simulink model "MBNLC_cascade_rov"  (Simulink 6.0)
settings: Solver=ode45  StartTime=0.0  StopTime=650  RelTol=1e-3
undefined symbols (not defined in the file): B, DQ, DQL, I, m, M, Ma, MaL, MaU, rg, sigbuilder_block, T, W, xb, xg, Xudot, yb, yg, Yvdot, zb, zg, Zwdot
libraries: simulink_extras x12, simulink x8
(part 1 of 3)
settings Model: LastModifiedBy=c chin

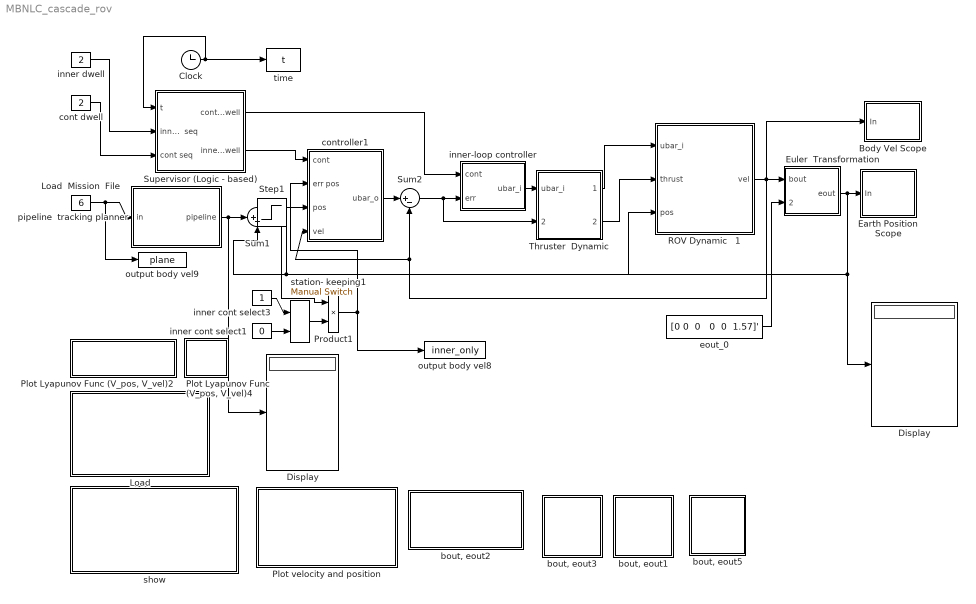
== system MBNLC_cascade_rov ==
  " Load  " : Subsystem  AncestorBlock=|
      | rov_design_analysis/ROV Controller
      | Design
      | Applications/ Load RRCROV2 parameters
      settings: OpenFcn=|
      | clc
      | cd c:\Matlab7\toolbox\rov_design_analysis\\mat_file ;
      | load rrcrovf;
      mask Display: disp('Double-click \n to \n Load the\n RRCROV\n parameters')
  " ROV Dynamic   1" : Subsystem
      mask Display:
      | disp('ROV')
      | image(imread('/rov_design_analysis/fig/ROVRRC2.jpg'));
      | color('white');port_label('input',1,'ubar_i')
      | color('white');port_label('input',2,'thrust')
      | color('white');port_label('input',3,'eout')
      | 
      | 
      | color('white');port_label('output',1,'vel')
  " inner dwell" : Constant  Value=2
  " station- keeping1" : simulink/Signal Routing/Manual Switch  sw=1  action=0
  Body Vel Scope : Subsystem  AncestorBlock=|
      | rov_design_analysis/ROV Controller
      | Design
      | Applications/1. Heading autopilot/Earth Position
      | Scope
      mask Display: disp('Body\nVelocity\nScope')
  Clock : Clock
      settings: Decimation=10
  Display : Display
  "Display  " : Display
  "Earth Position Scope " : Subsystem  AncestorBlock=|
      | rov_design_analysis/ROV Controller
      | Design
      | Applications/1. Heading autopilot/Earth Position
      | Scope
      mask Display: disp('Earth\nPosition\nScope')
  Euler  Transformation : Subsystem  AncestorBlock=rov_design_analysis/Scope Utilities/Euler Transformation
      mask Display: disp('Navigation \n Sensor')
  Load  Mission  File : Constant  Value=6
  "Plot Lyapunov Func (V_pos, V_vel)2" : Subsystem  AncestorBlock=|
      | rov_design_analysis/ROV Controller
      | Design
      | Applications/Plot velocity and position
      settings: OpenFcn=|
      | clc
      | close all
      mask Display: disp('Close All Figure')
  "Plot Lyapunov Func (V_pos, V_vel)4" : Subsystem  AncestorBlock=|
      | rov_design_analysis/ROV Controller
      | Design
      | Applications/Plot velocity and position
      settings: OpenFcn=|
      | clc
      | clear
      mask Display: disp('Clear')
  Plot velocity and position : Subsystem  AncestorBlock=|
      | rov_design_analysis/ROV Controller
      | Design
      | Applications/Plot velocity and position
      settings: OpenFcn=|
      | clc
      | cd c:\Matlab7\toolbox\rov_design_analysis\\m_file ;
      | run nonlin_resp6
      mask Display: disp('Double-click \n to \n Plot Velocity \n and \n Position')
  Product1 : Product  RndMeth=Zero
  Sum1 : Sum  Inputs=|+-  OutDataTypeMode=double  SaturateOnIntegerOverflow=on
  Sum2 : Sum  Inputs=|+-  OutDataTypeMode=double  SaturateOnIntegerOverflow=on
  Supervisor (Logic - based) : Subsystem
      mask Display: disp('Supervisor \n (Logic-based)')
  Thruster  Dynamic : Subsystem
      mask Display: disp('Thruster \n Dynamic')
  "bout, eout1" : Subsystem  AncestorBlock=|
      | rov_design_analysis/ROV Controller
      | Design
      | Applications/Plot velocity and position
      settings: OpenFcn=|
      | clc
      | cd c:\Matlab7\toolbox\rov_design_analysis\\m_file ;
      | figure
      | plot(eout(:,1),-eout(:,3))
      | xlabel('x')
      | ylabel('z')
      mask Display: disp('Plot \n XZ ')
  "bout, eout2" : Subsystem  AncestorBlock=|
      | rov_design_analysis/ROV Controller
      | Design
      | Applications/Plot velocity and position
      settings: OpenFcn=|
      | clc
      | cd c:\Matlab7\toolbox\rov_design_analysis\\m_file ;
      | figure
      | plot3(eout(:,1), eout(:,2),-eout(:,3))
      | xlabel('x')
      | ylabel('y')
      | zlabel('z')
      | grid on
      mask Display: disp('Plot \n 3D Response')
  "bout, eout3" : Subsystem  AncestorBlock=|
      | rov_design_analysis/ROV Controller
      | Design
      | Applications/Plot velocity and position
      settings: OpenFcn=|
      | clc
      | cd c:\Matlab7\toolbox\rov_design_analysis\\m_file ;
      | figure
      | plot(eout(:,1), eout(:,2))
      | xlabel('x')
      | ylabel('y')
      mask Display: disp('Plot \n XY ')
  "bout, eout5" : Subsystem  AncestorBlock=|
      | rov_design_analysis/ROV Controller
      | Design
      | Applications/Plot velocity and position
      settings: OpenFcn=|
      | clc
      | cd c:\Matlab7\toolbox\rov_design_analysis\\m_file ;
      | figure
      | box off
      | subplot(4,1,1)
      | plot(inner.time,inner.signals.values)
      | xlabel('time (sec)')
      | ylabel('Inner controller type')
      | subplot(4,1,2)
      | plot(outer.time,outer.signals.values)
      | xlabel('time (sec)')
      | ylabel('Outer controller type')
      | subplot(4,1,3)
      | plot(plane.time,plane.signals.values)
      | xlabel('time (sec)')
      | ylabel('Input sequence')
      | 
      | subplot(4,1,4)
      | plot(inner_only.time,inner_only.signals.values)
      | xlabel('time (sec)')
      | ylabel('Inner/Outer loop')
      mask Display: disp('Plot \n switching \n signal ')
  cont dwell : Constant  Value=2
  controller1 : Subsystem  Description=f(x)  AncestorBlock=|
      | rov_design_analysis/ROV Controller
      | Design
      | Applications/1. Heading autopilot/controller
      mask Display: disp('Nonlinear \n Model-Based \n Outer \n Controller')
  eout_0 : Constant  Value="[0 0  0   0  0  1.57]'"  OutDataTypeMode=double
  inner cont select1 : Constant  Value=0
  inner cont select3 : Constant
  inner-loop controller : Subsystem  Description=f(x)  AncestorBlock=|
      | rov_design_analysis/ROV Controller
      | Design
      | Applications/1. Heading autopilot/controller
      mask Display: disp('Inner Loop \n Controller')
  output body vel8 : ToWorkspace  VariableName=inner_only  SampleTime=1  SaveFormat=Structure With Time
  output body vel9 : ToWorkspace  VariableName=plane  SampleTime=1  SaveFormat=Structure With Time
  "pipeline  tracking planner  " : Subsystem  AncestorBlock=|
      | rov_design_analysis/ROV Controller
      | Design
      | Applications/1. Heading autopilot/pipe tracking
      | profile
      | (Auto)
      mask Display: disp('Pipeline Tracking \n Planner')
  show : Subsystem  AncestorBlock=|
      | rov_design_analysis/ROV Controller
      | Design
      | Applications/ Load RRCROV2 parameters
      settings: OpenFcn=|
      | clc
      | cd  c:\Matlab7\toolbox\rov_design_analysis\hybrid ;
      | open rrcrov2_para
      mask Display: disp('Double-click \n to \n SHOW\n RRCROV\n parameters')
  time : ToWorkspace  VariableName=t  SampleTime=1  SaveFormat=Array
  Step1 : Step  IOType=siggen  SampleTime=0
  wires:
  " ROV Dynamic   1"/1(vel) -> Body Vel Scope/1(In), Sum2/2, controller1/4(vel), Euler  Transformation/1(bout)
  Euler  Transformation/1(eout) -> "Earth Position Scope "/1(In), controller1/3(pos), Sum1/2, " ROV Dynamic   1"/3("pos "), "Display  "/1
  Clock/1 -> time/1, Supervisor (Logic - based)/1(t)
  Thruster  Dynamic/2(thruster_out) -> " ROV Dynamic   1"/2("thrust ")
  Sum2/1 -> Thruster  Dynamic/2(bout_err), inner-loop controller/2(err)
  Thruster  Dynamic/1(cont_out) -> " ROV Dynamic   1"/1(ubar_i)
  inner-loop controller/1(ubar_i) -> Thruster  Dynamic/1(ubar_i)
  "pipeline  tracking planner  "/1(pipeline) -> Sum1/1, Display/1
  Supervisor (Logic - based)/1(cont dwell) -> inner-loop controller/1(cont)
  controller1/1(ubar_o) -> Sum2/1
  " inner dwell"/1 -> Supervisor (Logic - based)/2(inner  seq)
  cont dwell/1 -> Supervisor (Logic - based)/3(cont seq)
  eout_0/1 -> Euler  Transformation/2(eout_0)
  Load  Mission  File/1 -> output body vel9/1, "pipeline  tracking planner  "/1(in)
  inner cont select3/1 -> " station- keeping1"/1
  inner cont select1/1 -> " station- keeping1"/2
  " station- keeping1"/1 -> Product1/2
  Sum1/1 -> Product1/1
  Supervisor (Logic - based)/2(inner  dwell) -> controller1/1(cont)
  Product1/1 -> controller1/2(err pos), output body vel8/1

== system MBNLC_cascade_rov/ Load   ==

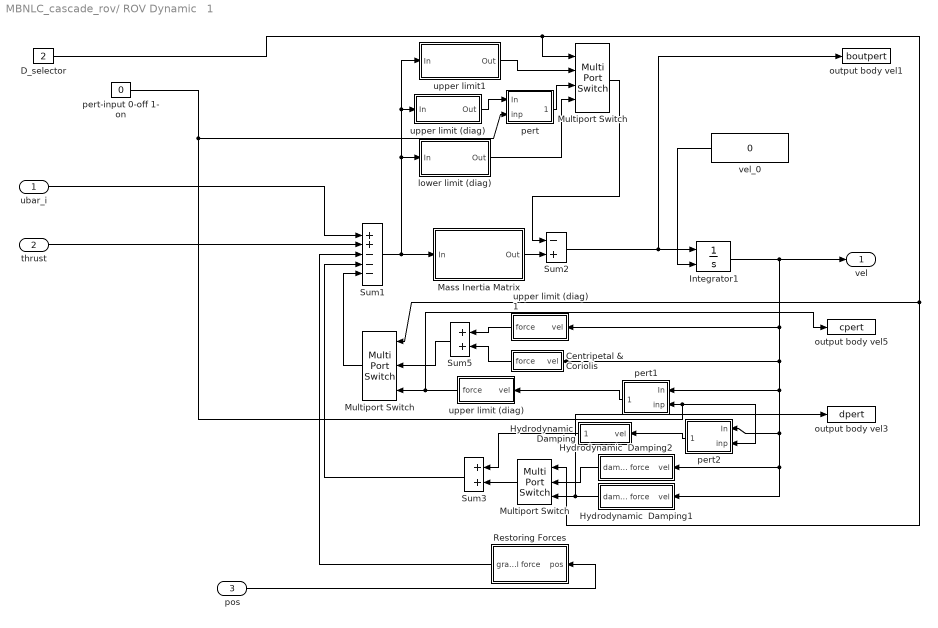
== system MBNLC_cascade_rov/ ROV Dynamic   1 ==
  ubar_i : Inport  Port=1  LatchInput=off
  "thrust " : Inport  Port=2  LatchInput=off
  "pos " : Inport  Port=3  LatchInput=off
  Centripetal & Coriolis : Subsystem  Orientation=left  AncestorBlock=rov_design_analysis/ROV Models/1. Six DOF RRC ROV II/Centripetal & Coriolis
      mask Display: disp('C')
  D_selector : Constant  Value=2
  Hydrodynamic  Damping : Subsystem  Orientation=left
      mask Display: disp('D')
  Hydrodynamic  Damping1 : Subsystem  Orientation=left
      mask Display: disp('perturb \nDamping')
  Hydrodynamic  Damping2 : Subsystem  Orientation=left
      mask Display: disp('Zero Perturb')
  Integrator1 : Integrator  InitialConditionSource=external
  Mass Inertia Matrix : Subsystem
      mask Display: disp('inv(MRB+MA)')
  Multiport Switch : MultiPortSwitch  Inputs=3
  "Multiport Switch  " : MultiPortSwitch  Orientation=left  Inputs=2
  "Multiport Switch    " : MultiPortSwitch  Orientation=left  Inputs=2
  Restoring Forces : Subsystem  Orientation=left
      mask Display: disp('Restoring\nForce')
  Sum1 : Sum  Inputs=++---  SaturateOnIntegerOverflow=on  InputSameDT=on
  Sum2 : Sum  Inputs=-+  SaturateOnIntegerOverflow=on  InputSameDT=on
  Sum3 : Sum  Orientation=left  SaturateOnIntegerOverflow=on  InputSameDT=on
  Sum5 : Sum  Orientation=left  SaturateOnIntegerOverflow=on  InputSameDT=on
  lower limit (diag) : Subsystem
      mask Display: disp('Perturb MA')
  output body vel1 : ToWorkspace  VariableName=boutpert  SampleTime=1  SaveFormat=Array
  output body vel3 : ToWorkspace  VariableName=dpert  SampleTime=1  SaveFormat=Array
  output body vel5 : ToWorkspace  VariableName=cpert  SampleTime=1  SaveFormat=Array
  pert : Subsystem
  pert-input 0-off 1- on : Constant  Value=0
  pert1 : Subsystem  Orientation=left
  pert2 : Subsystem  Orientation=left
  upper limit (diag) : Subsystem
      mask Display: disp('Perturb MA')
  "upper limit (diag)   " : Subsystem  Orientation=left
      mask Display: disp('Perturb CA')
  upper limit (diag)   1 : Subsystem  Orientation=left
      mask Display: disp('CA')
  upper limit1 : Subsystem
      mask Display: disp('Zero Perturb')
  vel_0 : Constant  Orientation=left  Value=0  OutDataTypeMode=double
  vel : Outport
  wires:
  Restoring Forces/1(gravitational force) -> Sum1/3
  "thrust "/1 -> Sum1/2
  Sum1/1 -> Mass Inertia Matrix/1(In), upper limit1/1(In), upper limit (diag)/1(In), lower limit (diag)/1(In)
  "Multiport Switch  "/1 -> Sum1/5
  "pos "/1 -> Restoring Forces/1(pos)
  Mass Inertia Matrix/1(Out) -> Sum2/2
  upper limit1/1(Out) -> Multiport Switch/2
  lower limit (diag)/1(Out) -> Multiport Switch/4
  Multiport Switch/1 -> Sum2/1
  "upper limit (diag)   "/1(force) -> "Multiport Switch  "/3, output body vel5/1
  Sum5/1 -> "Multiport Switch  "/2
  Hydrodynamic  Damping1/1(damping force) -> "Multiport Switch    "/3, output body vel3/1
  Hydrodynamic  Damping2/1(damping force) -> "Multiport Switch    "/2
  Sum3/1 -> Sum1/4
  "Multiport Switch    "/1 -> Sum3/2
  Hydrodynamic  Damping/1(damping force) -> Sum3/1
  upper limit (diag)   1/1(force) -> Sum5/1
  Centripetal & Coriolis/1(force) -> Sum5/2
  Sum2/1 -> output body vel1/1, Integrator1/1
  Integrator1/1 -> vel/1, upper limit (diag)   1/1(vel), Centripetal & Coriolis/1(vel), Hydrodynamic  Damping1/1(vel), Hydrodynamic  Damping2/1(vel), pert2/1(In), pert1/1(In)
  vel_0/1 -> Integrator1/2
  ubar_i/1 -> Sum1/1
  pert2/1(on/off) -> Hydrodynamic  Damping/1(vel)
  pert1/1(on/off) -> "upper limit (diag)   "/1(vel)
  upper limit (diag)/1(Out) -> pert/1(In)
  pert/1(on/off) -> Multiport Switch/3
  pert-input 0-off 1- on/1 -> pert/2(inp), pert1/2(inp), pert2/2(inp)
  D_selector/1 -> Multiport Switch/1, "Multiport Switch  "/1, "Multiport Switch    "/1

== system MBNLC_cascade_rov/Body Vel Scope ==
  In : Inport  Port=1  LatchInput=off
  Demux : Demux  Outputs=6
  output body vel4 : ToWorkspace  VariableName=bout  SampleTime=1  SaveFormat=Array
  phi : Scope
      settings: TickLabels=on  YMin=-0.125  YMax=0.2  DataFormat=Array
  theta : Scope
      settings: TickLabels=on  TimeRange=200  YMin=-0.05  YMax=0.15  DataFormat=Array
  x : Scope
      settings: TickLabels=on  TimeRange=50  YMin=-0.025  YMax=0.375  DataFormat=Array
  y : Scope
      settings: TickLabels=on  YMin=-0.02  YMax=0.1  DataFormat=Array
  yaw : Scope
      settings: TickLabels=on  TimeRange=200  YMin=-0.05  YMax=0.15  SaveName=ScopeData2  DataFormat=Array
  z : Scope
      settings: TickLabels=on  TimeRange=50  YMin=-0.0025  YMax=0.0375  DataFormat=Array
  wires:
  Demux/5 -> theta/1
  In/1 -> Demux/1, output body vel4/1
  Demux/3 -> z/1
  Demux/4 -> phi/1
  Demux/2 -> y/1
  Demux/1 -> x/1
  Demux/6 -> yaw/1

== system MBNLC_cascade_rov/Earth Position Scope  ==
  In : Inport  Port=1  LatchInput=off
  Demux : Demux  Outputs=6
  XY Graph : simulink/Sinks/XY Graph  xmin=-50  xmax=50  ymin=-50  ymax=50  st=-1
  output body vel5 : ToWorkspace  VariableName=eout  SampleTime=1  SaveFormat=Array
  phi : Scope
      settings: TickLabels=on  YMin=-0.125  YMax=0.2  DataFormat=Array
  theta : Scope
      settings: TickLabels=on  TimeRange=200  YMin=-0.05  YMax=0.15  DataFormat=Array
  x : Scope
      settings: TickLabels=on  TimeRange=50  YMin=-0.025  YMax=0.375  DataFormat=Array
  y : Scope
      settings: TickLabels=on  YMin=-0.02  YMax=0.1  DataFormat=Array
  yaw : Scope
      settings: TickLabels=on  TimeRange=200  YMin=-0.05  YMax=0.15  SaveName=ScopeData2  DataFormat=Array
  z : Scope
      settings: TickLabels=on  TimeRange=50  YMin=-0.0025  YMax=0.0375  DataFormat=Array
  wires:
  Demux/5 -> theta/1
  In/1 -> Demux/1, output body vel5/1
  Demux/3 -> z/1
  Demux/4 -> phi/1
  Demux/2 -> y/1, XY Graph/2
  Demux/1 -> x/1, XY Graph/1
  Demux/6 -> yaw/1

== system MBNLC_cascade_rov/Euler  Transformation ==
  bout : Inport  Port=1  LatchInput=off
  eout_0 : Inport  Port=2  LatchInput=off
  Demux : Demux  Outputs=2
  Demux1 : Demux  Outputs=2
  Intregrator2 : Integrator  InitialConditionSource=external
  Mux1 : Mux  Inputs=2
  Terminator : Terminator
  Transformation matrix R : Subsystem
      mask Display: disp('Transformation R')
  Transformation matrix T : Subsystem
      mask Display: disp('Transformation T')
  output body vel1 : ToWorkspace  VariableName=eoutpert  SampleTime=1  SaveFormat=Array
  eout : Outport  InitialOutput=0
  wires:
  Mux1/1 -> Intregrator2/1
  Intregrator2/1 -> Demux1/1, eout/1, output body vel1/1
  Demux/2 -> Transformation matrix R/1(angular body  velocity)
  Demux/1 -> Transformation matrix T/1(translational body velocity)
  bout/1 -> Demux/1
  Demux1/2 -> Transformation matrix T/2(angular position), Transformation matrix R/2(angular position)
  Transformation matrix R/1(angular earth velocity) -> Mux1/2
  Transformation matrix T/1(translational earth velocity) -> Mux1/1
  Demux1/1 -> Terminator/1
  eout_0/1 -> Intregrator2/2

== system MBNLC_cascade_rov/Plot Lyapunov Func (V_pos, V_vel)2 ==

== system MBNLC_cascade_rov/Plot Lyapunov Func (V_pos, V_vel)4 ==

== system MBNLC_cascade_rov/Plot velocity and position ==

== system MBNLC_cascade_rov/Supervisor (Logic - based) ==
  t : Inport  Port=1  LatchInput=off
  inner  seq : Inport  Port=2  LatchInput=off
  cont seq : Inport  Port=3  LatchInput=off
  150-300 : Relay  OnSwitchValue=150  OffSwitchValue=0  OnOutputValue=0  OffOutputValue=1
  Constant1 : Constant
  Constant8 : Constant
  Switching sequence : Subsystem  AncestorBlock=rov_design_analysis/Scope Utilities/Switching sequence
      mask Display: disp('Dwell \n Sequence')
  Switching sequence1 : Subsystem  AncestorBlock=rov_design_analysis/Scope Utilities/Switching sequence
      mask Display: disp('Dwell \n Sequence')
  "cont dwell switch  " : MultiPortSwitch  Inputs=2
  inner dwell Switch : MultiPortSwitch  Inputs=3
  output body vel6 : ToWorkspace  VariableName=outer  SampleTime=1  SaveFormat=Structure With Time
  cont dwell : Outport
  inner  dwell : Outport  Port=2
  wires:
  inner  seq/1 -> inner dwell Switch/1
  150-300/1 -> inner dwell Switch/2  "1"
  Constant8/1 -> inner dwell Switch/3  "2"
  inner dwell Switch/1 -> inner  dwell/1
  cont seq/1 -> "cont dwell switch  "/1
  "cont dwell switch  "/1 -> cont dwell/1, output body vel6/1
  t/1 -> 150-300/1
  Switching sequence1/1(" ") -> "cont dwell switch  "/2
  Constant1/1 -> "cont dwell switch  "/3
  Switching sequence/1(" ") -> inner dwell Switch/4  "3"

== system MBNLC_cascade_rov/Thruster  Dynamic ==
  ubar_i : Inport  Port=1  LatchInput=off
  bout_err : Inport  Port=2  LatchInput=off
  Sum2 : Sum  Inputs=|++  OutDataTypeMode=double  SaturateOnIntegerOverflow=on
  Thruster configuration1 : Subsystem  AncestorBlock=|
      | rov_design_analysis/ROV Controller
      | Design
      | Applications/1. Heading autopilot/Thruster
      | configuration
      mask Display: disp('T')
  Thruster configuration2 : Subsystem  AncestorBlock=|
      | rov_design_analysis/ROV Controller
      | Design
      | Applications/1. Heading autopilot/Thruster
      | configuration
      mask Display: disp('Kc')
  Thruster configuration3 : Subsystem  AncestorBlock=|
      | rov_design_analysis/ROV Controller
      | Design
      | Applications/1. Heading autopilot/Thruster
      | configuration
      mask Display: disp('Kc')
  Thruster configuration4 : Subsystem  AncestorBlock=|
      | rov_design_analysis/ROV Controller
      | Design
      | Applications/1. Heading autopilot/Thruster
      | configuration
      mask Display: disp('T')
  output earth pos1 : ToWorkspace  VariableName=thrustdc  SampleTime=1  SaveFormat=Array
  output earth pos2 : ToWorkspace  VariableName=thrustd  SampleTime=1  SaveFormat=Array
  output earth pos3 : ToWorkspace  VariableName=thrust  SampleTime=1  SaveFormat=Array
  thruster  dynamic     1 : Subsystem
  cont_out : Outport
  thruster_out : Outport  Port=2
  wires:
  Thruster configuration1/1(output force) -> Thruster configuration2/1(input velocity)
  Thruster configuration4/1(output force) -> Thruster configuration3/1(input velocity)
  thruster  dynamic     1/1(T) -> Thruster configuration1/1(input velocity), Sum2/2, output earth pos3/1
  bout_err/1 -> thruster  dynamic     1/1(volt)
  Thruster configuration3/1(output force) -> cont_out/1
  ubar_i/1 -> Thruster configuration4/1(input velocity), Sum2/1, output earth pos1/1
  Thruster configuration2/1(output force) -> thruster_out/1
  Sum2/1 -> output earth pos2/1

== system MBNLC_cascade_rov/bout, eout1 ==

== system MBNLC_cascade_rov/bout, eout2 ==

== system MBNLC_cascade_rov/bout, eout3 ==

== system MBNLC_cascade_rov/bout, eout5 ==

== system MBNLC_cascade_rov/controller1 ==
  cont : Inport  Port=1  LatchInput=off
  err pos : Inport  Port=2  LatchInput=off
  pos : Inport  Port=3  LatchInput=off
  vel : Inport  Port=4  LatchInput=off
  Multiport Switch : MultiPortSwitch  Inputs=2
  Nonlinear model based  PD controller : Subsystem
  PD : Subsystem
  "boutd  " : Constant  Value="[0 0  0   0  0  0]'"  OutDataTypeMode=double
  ubar_o : Outport
  wires:
  Multiport Switch/1 -> ubar_o/1
  cont/1 -> Multiport Switch/1
  "boutd  "/1 -> Nonlinear model based  PD controller/2(vel_d)
  Nonlinear model based  PD controller/1(" ") -> Multiport Switch/2
  PD/1(" ") -> Multiport Switch/3
  err pos/1 -> PD/1(err), Nonlinear model based  PD controller/1(errpos)
  pos/1 -> Nonlinear model based  PD controller/3(pos)
  vel/1 -> Nonlinear model based  PD controller/4(vel)

== system MBNLC_cascade_rov/inner-loop controller ==
  cont : Inport  Port=1  LatchInput=off
  err : Inport  Port=2  LatchInput=off
  MCD_selector : Constant  Value=2
  Multiport Switch : MultiPortSwitch
  "inner -PI-decouple " : Subsystem
  inner -backstepping : Subsystem
  inner-P : Subsystem
  inner-sliding : Subsystem
  output body vel7 : ToWorkspace  VariableName=inner  SampleTime=1  SaveFormat=Structure With Time
  ubar_i : Outport
  wires:
  Multiport Switch/1 -> ubar_i/1
  cont/1 -> Multiport Switch/1, output body vel7/1
  "inner -PI-decouple "/1(" ") -> Multiport Switch/2
  inner-P/1(" ") -> Multiport Switch/3
  err/1 -> inner-P/1(P), inner-sliding/1(sliding), inner -backstepping/1(err), "inner -PI-decouple "/1(err)
  inner -backstepping/1(" ") -> Multiport Switch/4
  inner-sliding/1(" ") -> Multiport Switch/5
  MCD_selector/1 -> inner -backstepping/2(M_select)

== system MBNLC_cascade_rov/pipeline  tracking planner   ==
  in : Inport  Port=1  LatchInput=off
  decoupled input : Subsystem
  pipeline : Outport
  wires:
  in/1 -> decoupled input/1(In1)
  decoupled input/1(Out1) -> pipeline/1

== system MBNLC_cascade_rov/show ==

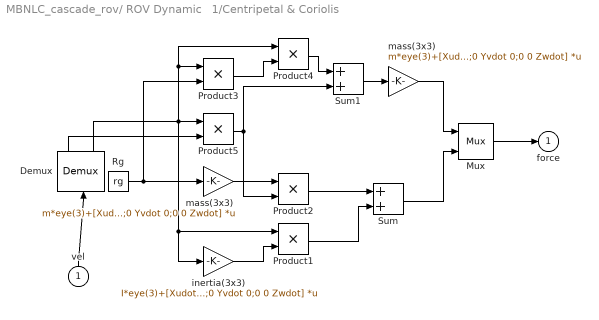
== system MBNLC_cascade_rov/ ROV Dynamic   1/Centripetal & Coriolis ==
  vel : Inport  Orientation=up  Port=1  LatchInput=off
  Demux : Demux  Orientation=up  Outputs=2
  Mux : Mux  Inputs=2
  Product{1..5} (5 alike) : Product  SaturateOnIntegerOverflow=on  RndMeth=Zero  InputSameDT=on
  Rg : Constant  Value=rg
  Sum : Sum  SaturateOnIntegerOverflow=on  InputSameDT=on
  Sum1 : Sum  SaturateOnIntegerOverflow=on  InputSameDT=on
  inertia(3x3) : Gain  Gain=I*eye(3)+[Xudot 0 0;0 Yvdot 0;0 0 Zwdot]  Multiplication=Matrix(K*u)  SaturateOnIntegerOverflow=on
  "mass(3x3) " : Gain  Gain=m*eye(3)+[Xudot 0 0;0 Yvdot 0;0 0 Zwdot]  Multiplication=Matrix(K*u)  SaturateOnIntegerOverflow=on
  "mass(3x3)   " : Gain  Gain=m*eye(3)+[Xudot 0 0;0 Yvdot 0;0 0 Zwdot]  Multiplication=Matrix(K*u)  SaturateOnIntegerOverflow=on
  force : Outport  InitialOutput=0
  wires:
  Product1/1 -> Sum/2
  "mass(3x3)   "/1 -> Product2/1
  Product2/1 -> Sum/1
  Rg/1 -> Product3/2, "mass(3x3)   "/1
  Product3/1 -> Product4/2
  Product4/1 -> Sum1/1
  Product5/1 -> Product2/2, Sum1/2
  Sum1/1 -> "mass(3x3) "/1
  Demux/2 -> Product5/1, Product3/1, Product4/1, Product1/1, inertia(3x3)/1
  Demux/1 -> Product5/2
  vel/1 -> Demux/1
  inertia(3x3)/1 -> Product1/2
  "mass(3x3) "/1 -> Mux/1
  Sum/1 -> Mux/2
  Mux/1 -> force/1

== system MBNLC_cascade_rov/ ROV Dynamic   1/Hydrodynamic  Damping ==
  vel : Inport  Port=1  LatchInput=off
  D linear : Gain  Gain=-diag(DQL)  SaturateOnIntegerOverflow=on
  damping force : Outport  InitialOutput=0
  wires:
  vel/1 -> D linear/1
  D linear/1 -> damping force/1

== system MBNLC_cascade_rov/ ROV Dynamic   1/Hydrodynamic  Damping1 ==
  vel : Inport  Port=1  LatchInput=off
  D quadratic : Gain  Gain=-diag(DQ)  SaturateOnIntegerOverflow=on
  Product : Product  SaturateOnIntegerOverflow=on  RndMeth=Zero  InputSameDT=on
  |u| : Abs  SaturateOnIntegerOverflow=on
  damping force : Outport  InitialOutput=0
  wires:
  Product/1 -> D quadratic/1
  vel/1 -> Product/1, |u|/1
  |u|/1 -> Product/2
  D quadratic/1 -> damping force/1

== system MBNLC_cascade_rov/ ROV Dynamic   1/Hydrodynamic  Damping2 ==
  vel : Inport  Port=1  LatchInput=off
  D quadratic : Gain  Gain=0  SaturateOnIntegerOverflow=on
  damping force : Outport  InitialOutput=0
  wires:
  D quadratic/1 -> damping force/1
  vel/1 -> D quadratic/1

== system MBNLC_cascade_rov/ ROV Dynamic   1/Mass Inertia Matrix ==
  In : Inport  Port=1  LatchInput=off
  inverse M : Gain  Gain=inv(M-Ma)  Multiplication=Matrix(K*u)  SaturateOnIntegerOverflow=on
  Out : Outport
  wires:
  inverse M/1 -> Out/1
  In/1 -> inverse M/1

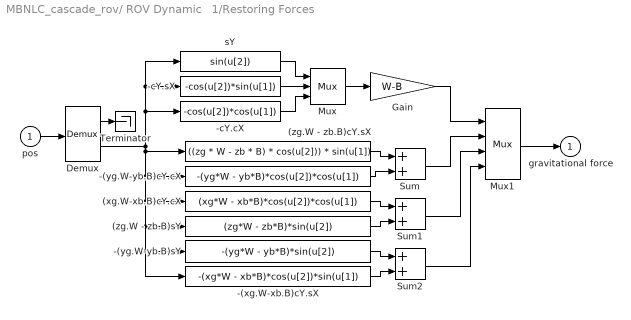
== system MBNLC_cascade_rov/ ROV Dynamic   1/Restoring Forces ==
  pos : Inport  Port=1  LatchInput=off
  (xg.W-xb.B)cY.cX : Fcn  Expr=(xg*W - xb*B)*cos(u[2])*cos(u[1])
  (zg.W - zb.B)cY.sX : Fcn  Expr=((zg * W - zb * B) * cos(u[2])) * sin(u[1])
  (zg.W - zb.B)sY : Fcn  Expr=(zg*W - zb*B)*sin(u[2])
  -(xg.W-xb.B)cY.sX : Fcn  Expr=-(xg*W - xb*B)*cos(u[2])*sin(u[1])
  -(yg.W-yb.B)cY.cX : Fcn  Expr=-(yg*W - yb*B)*cos(u[2])*cos(u[1])
  -(yg.W-yb.B)sY : Fcn  Expr=-(yg*W - yb*B)*sin(u[2])
  -cY.cX : Fcn  Expr=-cos(u[2])*cos(u[1])
  -cY.sX : Fcn  Expr=-cos(u[2])*sin(u[1])
  Demux : Demux  Outputs=2
  Gain : Gain  Gain=W-B  SaturateOnIntegerOverflow=on
  Mux : Mux  Inputs=3
  Mux1 : Mux
  Sum : Sum  SaturateOnIntegerOverflow=on  InputSameDT=on
  Sum1 : Sum  SaturateOnIntegerOverflow=on  InputSameDT=on
  Sum2 : Sum  SaturateOnIntegerOverflow=on  InputSameDT=on
  Terminator : Terminator
  sY : Fcn  Expr=sin(u[2])
  gravitational force : Outport  InitialOutput=0
  wires:
  Sum2/1 -> Mux1/4
  -(yg.W-yb.B)sY/1 -> Sum2/1
  -(xg.W-xb.B)cY.sX/1 -> Sum2/2
  Sum1/1 -> Mux1/3
  (xg.W-xb.B)cY.cX/1 -> Sum1/1
  (zg.W - zb.B)sY/1 -> Sum1/2
  Sum/1 -> Mux1/2
  (zg.W - zb.B)cY.sX/1 -> Sum/1
  -(yg.W-yb.B)cY.cX/1 -> Sum/2
  Gain/1 -> Mux1/1
  Mux/1 -> Gain/1
  -cY.cX/1 -> Mux/3
  -cY.sX/1 -> Mux/2
  sY/1 -> Mux/1
  Mux1/1 -> gravitational force/1
  Demux/2 -> -(xg.W-xb.B)cY.sX/1, -(yg.W-yb.B)sY/1, (zg.W - zb.B)sY/1, (xg.W-xb.B)cY.cX/1, -(yg.W-yb.B)cY.cX/1, (zg.W - zb.B)cY.sX/1, sY/1, -cY.sX/1, -cY.cX/1
  Demux/1 -> Terminator/1
  pos/1 -> Demux/1

== system MBNLC_cascade_rov/ ROV Dynamic   1/lower limit (diag) ==
  In : Inport  Port=1  LatchInput=off
  inverse M : Gain  Gain=-diag([21.1403-21.0981 51.7012-51.0026 92.451-91.837 3.6191-3.576 2.6427-2.7687 2.3033-2.3493])  Multiplication=Matrix(K*u)  SaturateOnIntegerOverflow=on
  Out : Outport
  wires:
  inverse M/1 -> Out/1
  In/1 -> inverse M/1

== system MBNLC_cascade_rov/ ROV Dynamic   1/pert ==
  In : Inport  Port=1  LatchInput=off
  inp : Inport  Port=2  LatchInput=off
  D linear3 : Gain  Gain=2  SaturateOnIntegerOverflow=on
  Product : Product  RndMeth=Zero
  Sine Wave-pert : Sin  Amplitude=0.1  SampleTime=0
  Sum6 : Sum  Inputs=|++  SaturateOnIntegerOverflow=on  InputSameDT=on
  on/off : Outport
  wires:
  D linear3/1 -> Sum6/1
  Sine Wave-pert/1 -> Product/1
  Product/1 -> Sum6/2
  inp/1 -> Product/2
  In/1 -> D linear3/1
  Sum6/1 -> on/off/1

== system MBNLC_cascade_rov/ ROV Dynamic   1/pert1 ==
  In : Inport  Port=1  LatchInput=off
  inp : Inport  Port=2  LatchInput=off
  D linear3 : Gain  Gain=2  SaturateOnIntegerOverflow=on
  Product : Product  RndMeth=Zero
  Sine Wave-pert : Sin  Amplitude=0.1  SampleTime=0
  Sum6 : Sum  Inputs=|++  SaturateOnIntegerOverflow=on  InputSameDT=on
  on/off : Outport
  wires:
  D linear3/1 -> Sum6/1
  Sine Wave-pert/1 -> Product/1
  Product/1 -> Sum6/2
  inp/1 -> Product/2
  In/1 -> D linear3/1
  Sum6/1 -> on/off/1

== system MBNLC_cascade_rov/ ROV Dynamic   1/pert2 ==
  In : Inport  Port=1  LatchInput=off
  inp : Inport  Port=2  LatchInput=off
  D linear3 : Gain  Gain=2  SaturateOnIntegerOverflow=on
  Product : Product  RndMeth=Zero
  Sine Wave-pert : Sin  Amplitude=0.1  SampleTime=0
  Sum6 : Sum  Inputs=|++  SaturateOnIntegerOverflow=on  InputSameDT=on
  on/off : Outport
  wires:
  D linear3/1 -> Sum6/1
  Sine Wave-pert/1 -> Product/1
  Product/1 -> Sum6/2
  inp/1 -> Product/2
  In/1 -> D linear3/1
  Sum6/1 -> on/off/1

== system MBNLC_cascade_rov/ ROV Dynamic   1/upper limit (diag) ==
  In : Inport  Port=1  LatchInput=off
  inverse M : Gain  Gain=-diag([21.724-21.1403 51.7013-51.7012 94.3-92.451 4.2176-3.6191 7.1148-2.6427 4.7673-2.3033])  Multiplication=Matrix(K*u)  SaturateOnIntegerOverflow=on
  Out : Outport
  wires:
  inverse M/1 -> Out/1
  In/1 -> inverse M/1

== system MBNLC_cascade_rov/ ROV Dynamic   1/upper limit (diag)    ==
  note: 7 8 9 10 11 12
  note: 1 2 3 4 5 6
  vel : Inport  Port=1  LatchInput=off
  (zg.W - zb.B)cY.sX : Fcn  Expr=-u[9]*u[3]*u[5]+u[8]*u[2]*u[6]
  (zg.W - zb.B)cY.sX1 : Fcn  Expr=u[9]*u[3]*u[4]-u[7]*u[1]*u[6]
  (zg.W - zb.B)cY.sX2 : Fcn  Expr=-u[8]*u[2]*u[4]+u[7]*u[1]*u[5]
  (zg.W - zb.B)cY.sX3 : Fcn  Expr=-u[9]*u[3]*u[2]+u[8]*u[2]*u[3]-u[12]*u[6]*u[5]+u[11]*u[5]*u[6]
  (zg.W - zb.B)cY.sX4 : Fcn  Expr=u[9]*u[3]*u[1]-u[7]*u[1]*u[3]+u[6]*u[12]*u[4]-u[4]*u[10]*u[6]
  (zg.W - zb.B)cY.sX5 : Fcn  Expr=-u[8]*u[2]*u[1]+u[7]*u[1]*u[2]-u[11]*u[5]*u[4]+u[10]*u[4]*u[5]
  Mux1 : Mux  Inputs=6
  Mux3 : Mux  Inputs=2
  Rg1 : Constant  Value="[MaU(1)  MaU(2)  MaU(3)  MaU(4)  MaU(5)  MaU(6) ]'"
  force : Outport
  wires:
  Mux1/1 -> force/1
  (zg.W - zb.B)cY.sX/1 -> Mux1/1
  (zg.W - zb.B)cY.sX1/1 -> Mux1/2
  (zg.W - zb.B)cY.sX2/1 -> Mux1/3
  (zg.W - zb.B)cY.sX3/1 -> Mux1/4
  (zg.W - zb.B)cY.sX4/1 -> Mux1/5
  (zg.W - zb.B)cY.sX5/1 -> Mux1/6
  vel/1 -> Mux3/1
  Rg1/1 -> Mux3/2
  Mux3/1 -> (zg.W - zb.B)cY.sX/1, (zg.W - zb.B)cY.sX1/1, (zg.W - zb.B)cY.sX4/1, (zg.W - zb.B)cY.sX5/1, (zg.W - zb.B)cY.sX3/1, (zg.W - zb.B)cY.sX2/1

== system MBNLC_cascade_rov/ ROV Dynamic   1/upper limit (diag)   1 ==
  note: 7 8 9 10 11 12
  note: 1 2 3 4 5 6
  vel : Inport  Port=1  LatchInput=off
  (zg.W - zb.B)cY.sX : Fcn  Expr=-u[9]*u[3]*u[5]+u[8]*u[2]*u[6]
  (zg.W - zb.B)cY.sX1 : Fcn  Expr=u[9]*u[3]*u[4]-u[7]*u[1]*u[6]
  (zg.W - zb.B)cY.sX2 : Fcn  Expr=-u[8]*u[2]*u[4]+u[7]*u[1]*u[5]
  (zg.W - zb.B)cY.sX3 : Fcn  Expr=-u[9]*u[3]*u[2]+u[8]*u[2]*u[3]-u[12]*u[6]*u[5]+u[11]*u[5]*u[6]
  (zg.W - zb.B)cY.sX4 : Fcn  Expr=u[9]*u[3]*u[1]-u[7]*u[1]*u[3]+u[6]*u[12]*u[4]-u[4]*u[10]*u[6]
  (zg.W - zb.B)cY.sX5 : Fcn  Expr=-u[8]*u[2]*u[1]+u[7]*u[1]*u[2]-u[11]*u[5]*u[4]+u[10]*u[4]*u[5]
  Mux1 : Mux  Inputs=6
  Mux3 : Mux  Inputs=2
  Rg1 : Constant  Value="[Ma(1)  Ma(2)  Ma(3)  Ma(4)  Ma(5)  Ma(6) ]'"
  force : Outport
  wires:
  Mux1/1 -> force/1
  (zg.W - zb.B)cY.sX/1 -> Mux1/1
  (zg.W - zb.B)cY.sX1/1 -> Mux1/2
  (zg.W - zb.B)cY.sX2/1 -> Mux1/3
  (zg.W - zb.B)cY.sX3/1 -> Mux1/4
  (zg.W - zb.B)cY.sX4/1 -> Mux1/5
  (zg.W - zb.B)cY.sX5/1 -> Mux1/6
  vel/1 -> Mux3/1
  Rg1/1 -> Mux3/2
  Mux3/1 -> (zg.W - zb.B)cY.sX/1, (zg.W - zb.B)cY.sX1/1, (zg.W - zb.B)cY.sX4/1, (zg.W - zb.B)cY.sX5/1, (zg.W - zb.B)cY.sX3/1, (zg.W - zb.B)cY.sX2/1

== system MBNLC_cascade_rov/ ROV Dynamic   1/upper limit1 ==
  In : Inport  Port=1  LatchInput=off
  inverse M : Gain  Gain=0  Multiplication=Matrix(K*u)  SaturateOnIntegerOverflow=on
  Out : Outport
  wires:
  inverse M/1 -> Out/1
  In/1 -> inverse M/1

== system MBNLC_cascade_rov/Euler  Transformation/Transformation matrix R ==
  angular body  velocity : Inport  Port=1  LatchInput=off
  angular position : Inport  Port=2  LatchInput=off
  Mux : Mux  Inputs=3
  Row1 of T : Subsystem
      mask Display: disp('Row 1')
  Row2 of T : Subsystem
      mask Display: disp('Row 2')
  Row3 of T : Subsystem
      mask Display: disp('Row 3')
  angular earth velocity : Outport
  wires:
  angular position/1 -> Row3 of T/2(angular position), Row1 of T/2(angular position), Row2 of T/2(angular position)
  Mux/1 -> angular earth velocity/1
  Row3 of T/1(angular earth velocity (row 3)) -> Mux/3
  Row2 of T/1(angular earth velocity (row 2)) -> Mux/2
  Row1 of T/1(angular earth velocity (row 1)) -> Mux/1
  angular body  velocity/1 -> Row3 of T/1("angular body velocity "), Row2 of T/1("angular body velocity "), Row1 of T/1(angular body  velocity)

== system MBNLC_cascade_rov/Euler  Transformation/Transformation matrix T ==
  translational body velocity : Inport  Port=1  LatchInput=off
  angular position : Inport  Port=2  LatchInput=off
  Mux : Mux  Inputs=3
  Row1 of R : Subsystem
      mask Display: disp('Row 1')
  Row2 of R : Subsystem
      mask Display: disp('Row 2')
  Row3 of R : Subsystem
      mask Display: disp('Row 3')
  translational earth velocity : Outport  InitialOutput=0
  wires:
  Mux/1 -> translational earth velocity/1
  Row3 of R/1(translational earth velocity (row 3)) -> Mux/3
  Row2 of R/1(translational earth velocity (row 2)) -> Mux/2
  Row1 of R/1(translational earth velocity (row 1)) -> Mux/1
  angular position/1 -> Row3 of R/2(angular position), Row1 of R/2(angular position), Row2 of R/2(angular position)
  translational body velocity/1 -> Row1 of R/1(translational body velocity), Row2 of R/1(translational body velocity), Row3 of R/1(translational body velocity)

== system MBNLC_cascade_rov/Supervisor (Logic - based)/Switching sequence ==
  Add2 : Sum  Inputs=+++++++  OutScaling=2^-10
  Signal Builder2 : Subsystem  Tag=STV Subsys  LoadFcn=sigbuilder_block('load');  StartFcn=sigbuilder_block('start');  StopFcn=sigbuilder_block('stop');  ClipboardFcn=sigbuilder_block('clipboard');  mask(Sigbuilder block){}
      mask help: Sigbuilder GUI
      mask init:
      | if ~strcmp(get_param(bdroot(gcbh),'SimulationStatus'),'stopped') tuvar = sigbuilder_block('maskInit'); end
      settings: CopyFcn=sigbuilder_block('copy');  DeleteFcn=sigbuilder_block('delete');  ModelCloseFcn=sigbuilder_block('modelClose');  PreSaveFcn=sigbuilder_block('preSave');  NameChangeFcn=sigbuilder_block('namechange');  OpenFcn=sigbuilder_block('open',[0 19.5 768 499.5 ]);  CloseFcn=sigbuilder_block('close');
      mask Display: plot(0,0,100,100,[10,10,40,40,10],[80,20,20,80,80],[40,10],[50,50], [40,27,10],[65,72,56],[40,25,25,10],[28,28,43,43]);
  " " : Outport
  wires:
  Add2/1 -> " "/1
  Signal Builder2/7(Signal 7) -> Add2/7
  Signal Builder2/6(Signal 6) -> Add2/6
  Signal Builder2/5(Signal 5) -> Add2/5
  Signal Builder2/4(Signal 4) -> Add2/4
  Signal Builder2/3(Signal 3) -> Add2/3
  Signal Builder2/2(Signal 2) -> Add2/2
  Signal Builder2/1(Signal 1) -> Add2/1

== system MBNLC_cascade_rov/Supervisor (Logic - based)/Switching sequence1 ==
  Add2 : Sum  Inputs=+++++++  OutScaling=2^-10
  Signal Builder2 : Subsystem  Tag=STV Subsys  LoadFcn=sigbuilder_block('load');  StartFcn=sigbuilder_block('start');  StopFcn=sigbuilder_block('stop');  ClipboardFcn=sigbuilder_block('clipboard');  mask(Sigbuilder block){}
      mask help: Sigbuilder GUI
      mask init:
      | if ~strcmp(get_param(bdroot(gcbh),'SimulationStatus'),'stopped') tuvar = sigbuilder_block('maskInit'); end
      settings: CopyFcn=sigbuilder_block('copy');  DeleteFcn=sigbuilder_block('delete');  ModelCloseFcn=sigbuilder_block('modelClose');  PreSaveFcn=sigbuilder_block('preSave');  NameChangeFcn=sigbuilder_block('namechange');  OpenFcn=sigbuilder_block('open',[0 19.5 768 499.5 ]);  CloseFcn=sigbuilder_block('close');
      mask Display: plot(0,0,100,100,[10,10,40,40,10],[80,20,20,80,80],[40,10],[50,50], [40,27,10],[65,72,56],[40,25,25,10],[28,28,43,43]);
  " " : Outport
  wires:
  Add2/1 -> " "/1
  Signal Builder2/7(Signal 7) -> Add2/7
  Signal Builder2/6(Signal 6) -> Add2/6
  Signal Builder2/5(Signal 5) -> Add2/5
  Signal Builder2/4(Signal 4) -> Add2/4
  Signal Builder2/3(Signal 3) -> Add2/3
  Signal Builder2/2(Signal 2) -> Add2/2
  Signal Builder2/1(Signal 1) -> Add2/1

== system MBNLC_cascade_rov/Thruster  Dynamic/Thruster configuration1 ==
  input velocity : Inport  Orientation=up  Port=1  LatchInput=off
  Thruster Matrix : Gain  Gain=T  Multiplication=Matrix(K*u)  SaturateOnIntegerOverflow=on
  output force : Outport  InitialOutput=0
  wires:
  input velocity/1 -> Thruster Matrix/1
  Thruster Matrix/1 -> output force/1

== system MBNLC_cascade_rov/Thruster  Dynamic/Thruster configuration2 ==
  input velocity : Inport  Orientation=up  Port=1  LatchInput=off
  Thruster Matrix : Gain  Gain=[eye(3) zeros(3,3);zeros(2,6); [0 0 0 0 0 1]]  Multiplication=Matrix(K*u)  SaturateOnIntegerOverflow=on
  output force : Outport  InitialOutput=0
  wires:
  input velocity/1 -> Thruster Matrix/1
  Thruster Matrix/1 -> output force/1

== system MBNLC_cascade_rov/Thruster  Dynamic/Thruster configuration3 ==
  input velocity : Inport  Orientation=up  Port=1  LatchInput=off
  Thruster Matrix : Gain  Gain=[eye(3) zeros(3,3);zeros(2,6); [0 0 0 0 0 1]]  Multiplication=Matrix(K*u)  SaturateOnIntegerOverflow=on
  output force : Outport  InitialOutput=0
  wires:
  input velocity/1 -> Thruster Matrix/1
  Thruster Matrix/1 -> output force/1

== system MBNLC_cascade_rov/Thruster  Dynamic/Thruster configuration4 ==
  input velocity : Inport  Orientation=up  Port=1  LatchInput=off
  Thruster Matrix : Gain  Gain=T  Multiplication=Matrix(K*u)  SaturateOnIntegerOverflow=on
  output force : Outport  InitialOutput=0
  wires:
  input velocity/1 -> Thruster Matrix/1
  Thruster Matrix/1 -> output force/1

== system MBNLC_cascade_rov/Thruster  Dynamic/thruster  dynamic     1 ==
  volt : Inport  Orientation=down  Port=1  LatchInput=off
  Gain2 : Gain  Gain=0.5  SaturateOnIntegerOverflow=on
  Saturation : Saturate  UpperLimit=70  LowerLimit=-70
  "thruster  alloc. " : Subsystem
  T : Outport
  wires:
  volt/1 -> "thruster  alloc. "/1(err)
  "thruster  alloc. "/1(u) -> Gain2/1
  Saturation/1 -> T/1
  Gain2/1 -> Saturation/1

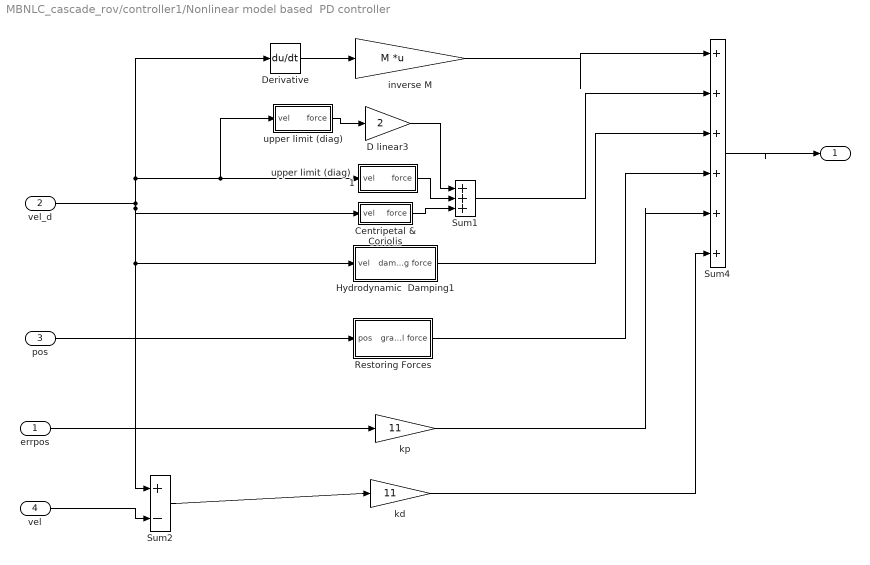
== system MBNLC_cascade_rov/controller1/Nonlinear model based  PD controller ==
  errpos : Inport  Port=1  LatchInput=off
  vel_d : Inport  Port=2  LatchInput=off
  pos : Inport  Port=3  LatchInput=off
  vel : Inport  Port=4  LatchInput=off
  Centripetal & Coriolis : Subsystem  AncestorBlock=rov_design_analysis/ROV Models/1. Six DOF RRC ROV II/Centripetal & Coriolis
      mask Display: disp('C')
  D linear3 : Gain  Gain=2  SaturateOnIntegerOverflow=on
  Derivative : Derivative
  Hydrodynamic  Damping1 : Subsystem
      mask Display: disp('Quadratic \nDamping')
  Restoring Forces : Subsystem
      mask Display: disp('Restoring\nForce')
  Sum1 : Sum  Inputs=+++  SaturateOnIntegerOverflow=on  InputSameDT=on
  Sum2 : Sum  Inputs=|+-  SaturateOnIntegerOverflow=on  InputSameDT=on
  Sum4 : Sum  Inputs=|++++++  SaturateOnIntegerOverflow=on  InputSameDT=on
  inverse M : Gain  Gain=M  Multiplication=Matrix(K*u)  SaturateOnIntegerOverflow=on
  "kd " : Gain  Gain=11  SaturateOnIntegerOverflow=on
  kp : Gain  Gain=11  SaturateOnIntegerOverflow=on
  "upper limit (diag)   " : Subsystem
      mask Display: disp('Perturb CA')
  upper limit (diag)   1 : Subsystem
      mask Display: disp('CA')
  " " : Outport
  wires:
  errpos/1 -> kp/1
  vel_d/1 -> Derivative/1, upper limit (diag)   1/1(vel), "upper limit (diag)   "/1(vel), Centripetal & Coriolis/1(vel), Hydrodynamic  Damping1/1(vel), Sum2/1
  Derivative/1 -> inverse M/1
  inverse M/1 -> Sum4/1
  Sum1/1 -> Sum4/2
  Hydrodynamic  Damping1/1(damping force) -> Sum4/3
  pos/1 -> Restoring Forces/1(pos)
  Restoring Forces/1(gravitational force) -> Sum4/4
  kp/1 -> Sum4/5
  Sum4/1 -> " "/1
  "kd "/1 -> Sum4/6
  vel/1 -> Sum2/2
  Sum2/1 -> "kd "/1
  Centripetal & Coriolis/1(force) -> Sum1/3
  upper limit (diag)   1/1(force) -> Sum1/2
  "upper limit (diag)   "/1(force) -> D linear3/1
  D linear3/1 -> Sum1/1

== system MBNLC_cascade_rov/controller1/PD ==
  err : Inport  Port=1  LatchInput=off
  Demux1 : Demux  Outputs=6
  Mux2 : Mux  Inputs=6
  PD Controller{1..4} (4 alike) : simulink_extras/Additional Linear/PID Controller  P=1  I=0  D=1
  " " : Outport
  wires:
  PD Controller3/1 -> Mux2/3
  err/1 -> Demux1/1
  Mux2/1 -> " "/1
  Demux1/1 -> PD Controller1/1
  PD Controller1/1 -> Mux2/1
  PD Controller2/1 -> Mux2/2
  PD Controller4/1 -> Mux2/6
  Demux1/2 -> PD Controller2/1
  Demux1/3 -> PD Controller3/1
  Demux1/6 -> PD Controller4/1

== system MBNLC_cascade_rov/inner-loop controller/inner -PI-decouple  ==
  err : Inport  Port=1  LatchInput=off
  Centripetal & Coriolis : Subsystem  AncestorBlock=rov_design_analysis/ROV Models/1. Six DOF RRC ROV II/Centripetal & Coriolis
      mask Display: disp('C')
  Gain2 : Gain  SaturateOnIntegerOverflow=on
  Hydrodynamic  Damping : Subsystem
      mask Display: disp('D')
  Hydrodynamic  Damping1 : Subsystem
      mask Display: disp('Perturb D')
  Sum : Sum  Inputs=|-++  SaturateOnIntegerOverflow=on  InputSameDT=on
  Sum1 : Sum  Inputs=+++  SaturateOnIntegerOverflow=on  InputSameDT=on
  Sum5 : Sum  Inputs=|++  SaturateOnIntegerOverflow=on  InputSameDT=on
  inner-PI : Subsystem
  "thruster  dynamic     " : Subsystem
  "upper limit (diag)   " : Subsystem
      mask Display: disp('Perturb CA')
  upper limit (diag)   1 : Subsystem
      mask Display: disp('CA')
  " " : Outport
  wires:
  err/1 -> upper limit (diag)   1/1(vel), Centripetal & Coriolis/1(vel), "upper limit (diag)   "/1(vel), Hydrodynamic  Damping/1(vel), Hydrodynamic  Damping1/1(vel), inner-PI/1(PI)
  upper limit (diag)   1/1(force) -> Sum1/1
  Centripetal & Coriolis/1(force) -> Sum1/2
  Hydrodynamic  Damping1/1(damping force) -> Sum5/2
  inner-PI/1(" ") -> Gain2/1
  "upper limit (diag)   "/1(force) -> Sum1/3
  Hydrodynamic  Damping/1(damping force) -> Sum5/1
  Gain2/1 -> Sum/1
  Sum5/1 -> Sum/3
  Sum1/1 -> Sum/2
  Sum/1 -> "thruster  dynamic     "/1(volt)
  "thruster  dynamic     "/1(T) -> " "/1

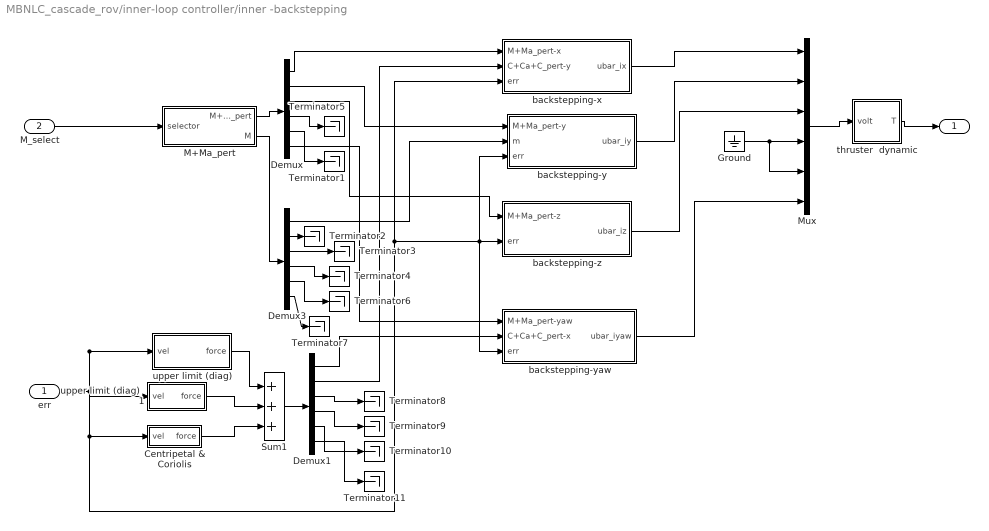
== system MBNLC_cascade_rov/inner-loop controller/inner -backstepping ==
  err : Inport  Port=1  LatchInput=off
  M_select : Inport  Port=2  LatchInput=off
  Centripetal & Coriolis : Subsystem  AncestorBlock=rov_design_analysis/ROV Models/1. Six DOF RRC ROV II/Centripetal & Coriolis
      mask Display: disp('C')
  Demux : Demux  Outputs=6
  Demux1 : Demux  Outputs=6
  Demux3 : Demux  Outputs=6
  Ground : Ground
  M+Ma_pert : Subsystem
  Mux : Mux  Inputs=6
  Sum1 : Sum  Inputs=+++  SaturateOnIntegerOverflow=on  InputSameDT=on
  Terminator{1..11} (11 alike) : Terminator
  backstepping-x : Subsystem
  backstepping-y : Subsystem
  backstepping-yaw : Subsystem
  backstepping-z : Subsystem
  "thruster  dynamic     " : Subsystem
  "upper limit (diag)   " : Subsystem
      mask Display: disp('Perturb CA')
  upper limit (diag)   1 : Subsystem
      mask Display: disp('CA')
  " " : Outport
  wires:
  M_select/1 -> M+Ma_pert/1(selector)
  err/1 -> "upper limit (diag)   "/1(vel), upper limit (diag)   1/1(vel), Centripetal & Coriolis/1(vel), backstepping-x/3(err), backstepping-y/3("err  "), backstepping-z/2("err  "), backstepping-yaw/3(err)
  M+Ma_pert/1(M+Ma_pert) -> Demux/1
  Centripetal & Coriolis/1(force) -> Sum1/3
  upper limit (diag)   1/1(force) -> Sum1/2
  "upper limit (diag)   "/1(force) -> Sum1/1
  Sum1/1 -> Demux1/1
  Demux/1 -> backstepping-x/1(M+Ma_pert-x)
  Demux1/2 -> backstepping-x/2(C+Ca+C_pert-y)
  Mux/1 -> "thruster  dynamic     "/1(volt)
  M+Ma_pert/2("M ") -> Demux3/1
  Demux3/1 -> backstepping-y/2(m)
  Demux/2 -> backstepping-y/1(M+Ma_pert-y)
  Demux/6 -> backstepping-yaw/1(M+Ma_pert-yaw)
  Demux1/1 -> backstepping-yaw/2(C+Ca+C_pert-x)
  Demux/3 -> backstepping-z/1(M+Ma_pert-z)
  backstepping-x/1(ubar_ix) -> Mux/1
  backstepping-y/1(ubar_iy) -> Mux/2
  backstepping-z/1(ubar_iz) -> Mux/3
  backstepping-yaw/1(ubar_iyaw) -> Mux/6
  Ground/1 -> Mux/4, Mux/5
  Demux/4 -> Terminator5/1
  Demux/5 -> Terminator1/1
  Demux3/2 -> Terminator2/1
  Demux3/3 -> Terminator3/1
  Demux3/4 -> Terminator4/1
  Demux3/5 -> Terminator6/1
  Demux3/6 -> Terminator7/1
  Demux1/3 -> Terminator8/1
  Demux1/4 -> Terminator9/1
  Demux1/5 -> Terminator10/1
  Demux1/6 -> Terminator11/1
  "thruster  dynamic     "/1(T) -> " "/1

== system MBNLC_cascade_rov/inner-loop controller/inner-P ==
  P : Inport  Port=1  LatchInput=off
  Demux1 : Demux
  Ground : Ground
  Mux2 : Mux  Inputs=6
  P Controller{1..4} (4 alike) : simulink_extras/Additional Linear/PID Controller  P=1  I=0  D=0
  Selector : Selector  Elements=[1 2 3 6]  InputPortWidth=6
  "thruster  dynamic     " : Subsystem
  " " : Outport
  wires:
  P Controller3/1 -> Mux2/3
  P Controller1/1 -> Mux2/1
  P Controller2/1 -> Mux2/2
  Selector/1 -> Demux1/1
  Demux1/1 -> P Controller1/1
  Demux1/2 -> P Controller2/1
  Demux1/3 -> P Controller3/1
  Demux1/4 -> P Controller4/1
  P Controller4/1 -> Mux2/6
  Ground/1 -> Mux2/4, Mux2/5
  P/1 -> Selector/1
  Mux2/1 -> "thruster  dynamic     "/1(volt)
  "thruster  dynamic     "/1(T) -> " "/1

== system MBNLC_cascade_rov/inner-loop controller/inner-sliding ==
  sliding : Inport  Port=1  LatchInput=off
  Sign : Signum
  "thruster  dynamic     " : Subsystem
  " " : Outport
  wires:
  Sign/1 -> "thruster  dynamic     "/1(volt)
  sliding/1 -> Sign/1
  "thruster  dynamic     "/1(T) -> " "/1

== system MBNLC_cascade_rov/pipeline  tracking planner  /decoupled input ==
  In1 : Inport  Orientation=down  Port=1  LatchInput=off
  relative pt : MultiPortSwitch  Inputs=8
  "x25, y=0, z=50 yaw=1.57" : Subsystem
  "x=0,y=0, z=0 yaw=0  " : Subsystem
  "x=15,y=0, z=45 yaw=0 " : Subsystem
  "x=25, z=45 yaw=0" : Subsystem
  "x=25,y=0, z=50 yaw=0" : Subsystem
  "x=25,y=40, z=50 yaw=0" : Subsystem
  "x=y=0, z=-50 yaw=0  " : Subsystem
  "x=y=15, z=50 yaw=0 " : Subsystem
  Out1 : Outport
  wires:
  "x=y=0, z=-50 yaw=0  "/1("1 ") -> relative pt/2  "1"
  "x=y=15, z=50 yaw=0 "/1(2) -> relative pt/3  "2"
  "x=15,y=0, z=45 yaw=0 "/1(3) -> relative pt/4  "3"
  "x=25, z=45 yaw=0"/1(4) -> relative pt/5  "4"
  "x=25,y=0, z=50 yaw=0"/1(5) -> relative pt/6  "5"
  "x25, y=0, z=50 yaw=1.57"/1(6) -> relative pt/7  "6"
  "x=25,y=40, z=50 yaw=0"/1(7) -> relative pt/8  "7"
  "x=0,y=0, z=0 yaw=0  "/1(8) -> relative pt/9  "8"
  In1/1 -> relative pt/1
  relative pt/1 -> Out1/1

== system MBNLC_cascade_rov/Euler  Transformation/Transformation matrix R/Row1 of T ==
  angular body  velocity : Inport  Port=1  LatchInput=off
  angular position : Inport  Port=2  LatchInput=off
  1 : Fcn  Expr=1
  Dot Product1 : simulink/Math Operations/Dot Product  InputSameDT=on  OutDataType=sfix(16)  OutScaling=2^-10  DoSatur=off
  Mux1 : Mux  Inputs=3
  cX.tY : Fcn  Expr=cos(u[1])*tan(u[2])
  sX.tY : Fcn  Expr=sin(u[1])*tan(u[2])
  angular earth velocity (row 1) : Outport
  wires:
  Dot Product1/1 -> angular earth velocity (row 1)/1
  angular body  velocity/1 -> Dot Product1/2
  Mux1/1 -> Dot Product1/1
  cX.tY/1 -> Mux1/3
  sX.tY/1 -> Mux1/2
  1/1 -> Mux1/1
  angular position/1 -> cX.tY/1, sX.tY/1, 1/1

== system MBNLC_cascade_rov/Euler  Transformation/Transformation matrix R/Row2 of T ==
  "angular body velocity " : Inport  Port=1  LatchInput=off
  angular position : Inport  Port=2  LatchInput=off
  -sX : Fcn  Expr=-sin(u[1])
  0 : Fcn  Expr=0
  Dot Product1 : simulink/Math Operations/Dot Product  InputSameDT=on  OutDataType=sfix(16)  OutScaling=2^-10  DoSatur=off
  Mux1 : Mux  Inputs=3
  cX : Fcn  Expr=cos(u[1])
  angular earth velocity (row 2) : Outport
  wires:
  Dot Product1/1 -> angular earth velocity (row 2)/1
  "angular body velocity "/1 -> Dot Product1/2
  Mux1/1 -> Dot Product1/1
  -sX/1 -> Mux1/3
  cX/1 -> Mux1/2
  0/1 -> Mux1/1
  angular position/1 -> -sX/1, cX/1, 0/1

== system MBNLC_cascade_rov/Euler  Transformation/Transformation matrix R/Row3 of T ==
  "angular body velocity " : Inport  Port=1  LatchInput=off
  angular position : Inport  Port=2  LatchInput=off
  1 : Fcn  Expr=0
  Dot Product1 : simulink/Math Operations/Dot Product  InputSameDT=on  OutDataType=sfix(16)  OutScaling=2^-10  DoSatur=off
  Mux1 : Mux  Inputs=3
  cX/cY : Fcn  Expr=cos(u[1])/cos(u[2])
  sX/cY : Fcn  Expr=sin(u[1])/cos(u[2])
  angular earth velocity (row 3) : Outport
  wires:
  Dot Product1/1 -> angular earth velocity (row 3)/1
  "angular body velocity "/1 -> Dot Product1/2
  Mux1/1 -> Dot Product1/1
  cX/cY/1 -> Mux1/3
  sX/cY/1 -> Mux1/2
  1/1 -> Mux1/1
  angular position/1 -> cX/cY/1, sX/cY/1, 1/1

== system MBNLC_cascade_rov/Euler  Transformation/Transformation matrix T/Row1 of R ==
  translational body velocity : Inport  Port=1  LatchInput=off
  angular position : Inport  Port=2  LatchInput=off
  -sZ.cX+cZ.sY.sX : Fcn  Expr=-sin(u[3])*cos(u[1]) + cos(u[3])*sin(u[2])*sin(u[1])
  Dot Product : simulink/Math Operations/Dot Product  InputSameDT=on  OutDataType=sfix(16)  OutScaling=2^-10  DoSatur=off
  Mux : Mux  Inputs=3
  cY.cZ : Fcn  Expr=cos(u[3]) * cos(u[2])
  sZ.sX+cZ.cX.sY : Fcn  Expr=sin(u[3])*sin(u[1]) + cos(u[3])*cos(u[1])*sin(u[2])
  translational earth velocity (row 1) : Outport
  wires:
  Dot Product/1 -> translational earth velocity (row 1)/1
  translational body velocity/1 -> Dot Product/2
  Mux/1 -> Dot Product/1
  sZ.sX+cZ.cX.sY/1 -> Mux/3
  -sZ.cX+cZ.sY.sX/1 -> Mux/2
  cY.cZ/1 -> Mux/1
  angular position/1 -> sZ.sX+cZ.cX.sY/1, -sZ.cX+cZ.sY.sX/1, cY.cZ/1

== system MBNLC_cascade_rov/Euler  Transformation/Transformation matrix T/Row2 of R ==
  translational body velocity : Inport  Port=1  LatchInput=off
  angular position : Inport  Port=2  LatchInput=off
  -cZ.sX+sY.sZ.cX : Fcn  Expr=-cos(u[3])*sin(u[1]) + sin(u[2])*sin(u[3])*cos(u[1])
  Dot Product1 : simulink/Math Operations/Dot Product  InputSameDT=on  OutDataType=sfix(16)  OutScaling=2^-10  DoSatur=off
  Mux1 : Mux  Inputs=3
  cY.sZ : Fcn  Expr=sin(u[3]) * cos(u[2])
  cZ.cX+sX.sY.sZ : Fcn  Expr=cos(u[3])*cos(u[1]) + sin(u[1])*sin(u[2])*sin(u[3])
  translational earth velocity (row 2) : Outport
  wires:
  Dot Product1/1 -> translational earth velocity (row 2)/1
  translational body velocity/1 -> Dot Product1/2
  Mux1/1 -> Dot Product1/1
  -cZ.sX+sY.sZ.cX/1 -> Mux1/3
  cZ.cX+sX.sY.sZ/1 -> Mux1/2
  cY.sZ/1 -> Mux1/1
  angular position/1 -> -cZ.sX+sY.sZ.cX/1, cZ.cX+sX.sY.sZ/1, cY.sZ/1

== system MBNLC_cascade_rov/Euler  Transformation/Transformation matrix T/Row3 of R ==
  translational body velocity : Inport  Port=1  LatchInput=off
  angular position : Inport  Port=2  LatchInput=off
  -sY : Fcn  Expr=-sin(u[2])
  Dot Product1 : simulink/Math Operations/Dot Product  InputSameDT=on  OutDataType=sfix(16)  OutScaling=2^-10  DoSatur=off
  Mux1 : Mux  Inputs=3
  cY.cX : Fcn  Expr=cos(u[2])*cos(u[1])
  cY.sX : Fcn  Expr=cos(u[2])*sin(u[1])
  translational earth velocity (row 3) : Outport  InitialOutput=0
  wires:
  Dot Product1/1 -> translational earth velocity (row 3)/1
  translational body velocity/1 -> Dot Product1/2
  Mux1/1 -> Dot Product1/1
  cY.cX/1 -> Mux1/3
  cY.sX/1 -> Mux1/2
  -sY/1 -> Mux1/1
  angular position/1 -> cY.cX/1, cY.sX/1, -sY/1

== system MBNLC_cascade_rov/Supervisor (Logic - based)/Switching sequence/Signal Builder2 ==
  Demux : Demux  Tag=STV Demux  Outputs=7
  FromWs : FromWorkspace  Tag=STV FromWs  VariableName=tuvar  SampleTime=0  SigBuilderData=DataTag0  VnvData=DataTag1
      SigBuilderData=|
      | channels(1).label = 'Signal 1'
      | channels(1).allXData = {[0 65 65 700]}
      | channels(1).allYData = {[1 1 0 0]}
      | channels(2).label = 'Signal 2'
      | channels(2).allXData = {[0 70 70 150 150 700]}
      | channels(2).allYData = {[0 0 1 1 0 0]}
      | channels(3).label = 'Signal 3'
      | channels(3).allXData = {[0 160 160 230 230 700]}
      | channels(3).allYData = {[0 0 1 1 0 0]}
      | channels(4).label = 'Signal 4'
      | channels(4).allXData = {[0 240 240 290 290 700]}
      | channels(4).allYData = {[0 0 1 1 0 0]}
      | channels(5).label = 'Signal 5'
      | channels(5).allXData = {[0 300 300 350 350 700]}
      | channels(5).allYData = {[0 0 1 1 0 0]}
      | channels(6).label = 'Signal 6'
      | channels(6).allXData = {[0 360 360 400 400 700]}
      | channels(6).allYData = {[0 0 1 1 0 0]}
      | channels(7).label = 'Signal 7'
      | channels(7).allXData = {[0 410 410 548 548 700]}
      | channels(7).allYData = {[0 0 1 1 0 0]}
      | dataSet.timeRange = [0 700]
      | dataSet.name = 'Group 1'
  Signal 1 : Outport  Tag=STV Outport
  Signal 2 : Outport  Tag=STV Outport  Port=2
  Signal 3 : Outport  Tag=STV Outport  Port=3
  Signal 4 : Outport  Tag=STV Outport  Port=4
  Signal 5 : Outport  Tag=STV Outport  Port=5
  Signal 6 : Outport  Tag=STV Outport  Port=6
  Signal 7 : Outport  Tag=STV Outport  Port=7
  wires:
  Demux/7 -> Signal 7/1
  Demux/6 -> Signal 6/1
  Demux/5 -> Signal 5/1
  Demux/4 -> Signal 4/1
  Demux/3 -> Signal 3/1
  Demux/2 -> Signal 2/1
  FromWs/1 -> Demux/1
  Demux/1 -> Signal 1/1
